simulink model "TASK_3"  (R2018b)
settings: Solver=VariableStepAuto  StartTime=0.0  StopTime=10.0  RelTol=1e-3
libraries: dspindex x1
settings Model: Creator=STUDENT  LastModifiedBy=Федор
settings SFSimCC: SimUseLocalCustomCode=off
settings RTWCC: RTWUseLocalCustomCode=off
settings CodeAppCC: StateflowObjectComments=on

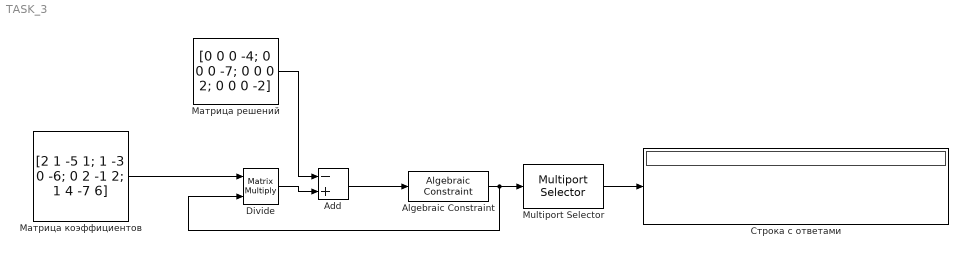
== system TASK_3 ==
  Add : Sum  Inputs=-+
  Algebraic Constraint : AlgebraicConstraint
  Divide : Product  Inputs=**  Multiplication=Matrix(*)
  Multiport Selector : dspindex/Multiport Selector  rowsOrCols=Columns  idxCellArray={4}  idxErrMode=Clip Index
  Матрица коэффициентов : Constant  Value=[2 1 -5 1; 1 -3 0 -6; 0 2 -1 2; 1 4 -7 6]
  Матрица решений : Constant  Value=[0 0 0 -4; 0 0 0 -7; 0 0 0 2; 0 0 0 -2]
  Строка с ответами : Display
  wires:
  Algebraic Constraint/1 -> Multiport Selector/1, Divide/2
  Матрица коэффициентов/1 -> Divide/1
  Divide/1 -> Add/2
  Add/1 -> Algebraic Constraint/1
  Матрица решений/1 -> Add/1
  Multiport Selector/1 -> Строка с ответами/1
